simulink model "Camera_Sensor_CS2017_Model_Template"  (Simulink 8.8)
settings: Solver=ode45  StartTime=0  StopTime=10  FixedStep=0.001  RelTol=1e-3  AbsTol=1e-6
libraries: Solver_SF x2
settings Model: Creator=ywata  LastModifiedBy=mkhan  ExtModeTrigMode=oneshot  ExtModeArmWhenConnect=off
settings DataIOCC: LimitDataPoints=off  SignalLoggingName=sigsOut
settings OptimizationCC: BlockReduction=off  BooleanDataType=off
settings DebuggingCC: SaveWithParameterizedLinksMsg=none  SignalResolutionControl=TryResolveAllWithWarning  MultiTaskDSMMsg=warning  MultiTaskCondExecSysMsg=none  SFExecutionAtInitializationDiag=warning
settings HardwareCC: TargetUnknown=on
settings RTWCC: TemplateMakefile=grt_vc.tmf
settings GRTTargetCC: TargetFcnLib=ansi_tfl_tmw.mat

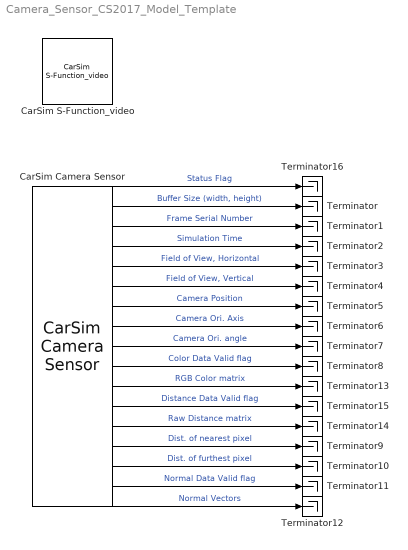
== system Camera_Sensor_CS2017_Model_Template ==
  CarSim Camera Sensor : Solver_SF/CarSim Camera Sensor  Priority=1  BufferName=EBS
  CarSim S-Function_video : Solver_SF/CarSim S-Function_video  Priority=1  SIMFILE=simfile.sim
  Terminator{,1..16} (17 alike) : Terminator
  wires:
  CarSim Camera Sensor/11 -> Terminator13/1  "RGB Color matrix"
  CarSim Camera Sensor/1 -> Terminator16/1  "Status Flag"
  CarSim Camera Sensor/13 -> Terminator14/1  "Raw Distance matrix"
  CarSim Camera Sensor/17 -> Terminator12/1  "Normal Vectors"
  CarSim Camera Sensor/2 -> Terminator/1  "Buffer Size (width, height)"
  CarSim Camera Sensor/14 -> Terminator9/1  "Dist. of nearest pixel"
  CarSim Camera Sensor/15 -> Terminator10/1  "Dist. of furthest pixel"
  CarSim Camera Sensor/16 -> Terminator11/1  "Normal Data Valid flag"
  CarSim Camera Sensor/12 -> Terminator15/1  "Distance Data Valid flag"
  CarSim Camera Sensor/10 -> Terminator8/1  "Color Data Valid flag"
  CarSim Camera Sensor/3 -> Terminator1/1  "Frame Serial Number"
  CarSim Camera Sensor/4 -> Terminator2/1  "Simulation Time"
  CarSim Camera Sensor/5 -> Terminator3/1  "Field of View, Horizontal"
  CarSim Camera Sensor/6 -> Terminator4/1  "Field of View, Vertical"
  CarSim Camera Sensor/7 -> Terminator5/1  "Camera Position"
  CarSim Camera Sensor/8 -> Terminator6/1  "Camera Ori. Axis"
  CarSim Camera Sensor/9 -> Terminator7/1  "Camera Ori. angle"
